simulink model "simulink_trot_continu"  (R2023a)
settings: Solver=VariableStepAuto  StartTime=0.0  StopTime=1.2  RelTol=1e-3
values from neighbouring files (symbols this model uses):
  denum_filtre = denum_ordre1    [Script_BE.m]
  Gain_Capteur = Gain_LEM    (= 0.104)    [Script_BE.m]
  K_Corr = K_LEM    (= 0.503460361152)    [Script_BE.m]
  L = 2*10^-3    (= 0.002)    [Script_BE.m]
  num_filtre = num_ordre1    [Script_BE.m]
  tau_i = tau_i_lem    (= 0.00397250737957)    [Script_BE.m]
  U_bat = 24    [Script_BE.m]
settings Model: Creator=bogen  LastModifiedBy=bogen

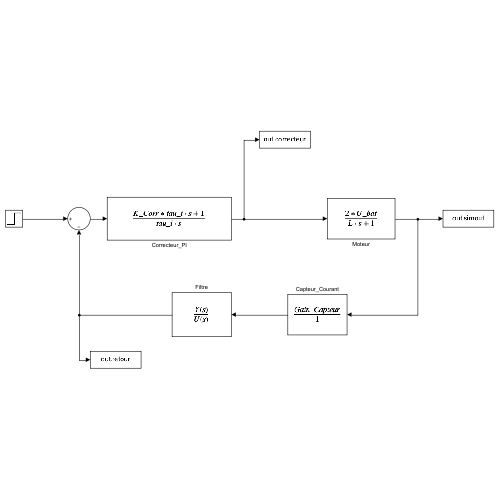
[thumbnail: Simulink's stored preview of the top-level diagram]
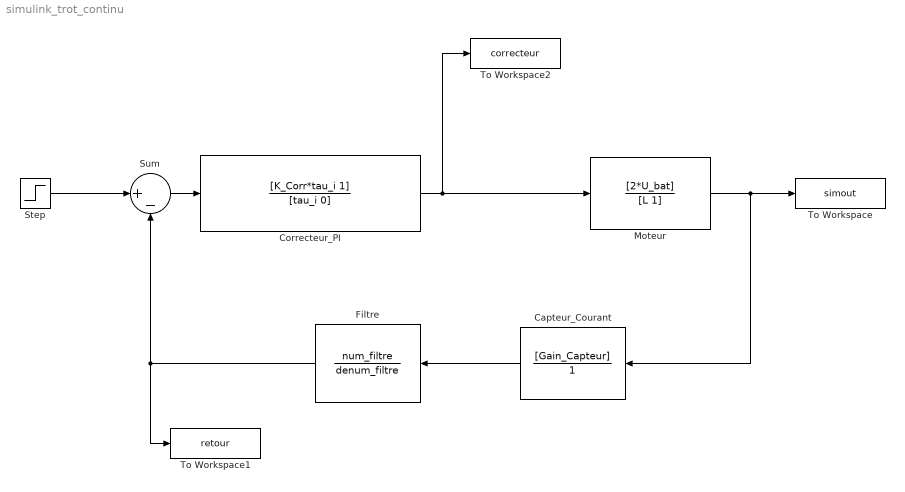
== system simulink_trot_continu ==
  Capteur_Courant : TransferFcn  Numerator=[Gain_Capteur]  Denominator=[1]
  Correcteur_PI : TransferFcn  Numerator=[K_Corr*tau_i 1]  Denominator=[tau_i 0]
  Filtre : TransferFcn  Numerator=num_filtre  Denominator=denum_filtre
  Moteur : TransferFcn  Numerator=[2*U_bat]  Denominator=[L 1]
  Step : Step  After=3.3  SampleTime=0
  Sum : Sum  Inputs=|+-
  To Workspace : ToWorkspace  VariableName=simout  SaveFormat=Timeseries  SampleTime=-1
  To Workspace1 : ToWorkspace  VariableName=retour  SaveFormat=Timeseries  SampleTime=-1
  To Workspace2 : ToWorkspace  VariableName=correcteur  SaveFormat=Timeseries  SampleTime=-1
  wires:
  Correcteur_PI/1 -> Moteur/1, To Workspace2/1
  Moteur/1 -> Capteur_Courant/1, To Workspace/1
  Capteur_Courant/1 -> Filtre/1
  Filtre/1 -> To Workspace1/1, Sum/2
  Step/1 -> Sum/1
  Sum/1 -> Correcteur_PI/1
